simulink library "TerryBodyBlockLib2G"  (R2018a)
settings: Solver=ode45  StartTime=0.0  StopTime=10.0  RelTol=1e-3  EnableMultiTasking=on
undefined symbols (not defined in the file): BaseMass, E, ExtendedActuatorLength, FollowerMass, H, L, N, rho, W, X, Y, Z
libraries: sm_lib x270, nesl_utility x94, fl_lib x18, simulink x2
(part 1 of 6)
settings Model: Creator=tdenery  LastModifiedBy=tdenery
settings DataIOCC: LimitDataPoints=on  SaveFormat=Array  SignalLoggingSaveFormat=ModelDataLogs
settings OptimizationCC: ExpressionDepthLimit=2147483647  LifeSpan=inf
settings DebuggingCC: UnderspecifiedInitializationDetection=Classic  MergeDetectMultiDrivingBlocksExec=none  SolverPrmCheckMsg=warning  FcnCallInpInsideContextMsg=warning  StateNameClashWarn=warning  SFUnexpectedBacktrackingDiag=warning  SFNoUnconditionalDefaultTransitionDiag=warning  SFExecutionAtInitializationDiag=none
settings HardwareCC: ProdBitPerPointer=32  ProdBitPerSizeT=32  ProdBitPerPtrDiffT=32  ProdLargestAtomicFloat=None  ProdIntDivRoundTo=Undefined  ProdEndianess=Unspecified  ProdWordSize=32  ProdHWDeviceType=32-bit Generic
settings ModelReferenceCC: PropagateSignalLabelsOutOfModel=off
settings CodeAppCC: StateflowObjectComments=on
settings GRTTargetCC: TargetLangStandard=C89/C90 (ANSI)  GeneratePreprocessorConditionals=Disable all  CombineOutputUpdateFcns=off  GRTInterface=on
settings ConfigComp: CovMetricSettings=dw  CovHtmlReporting=on  CovSaveCumulativeToWorkspaceVar=on  CovSaveSingleToWorkspaceVar=on  CovExternalEMLEnable=off  CovSFcnEnable=off

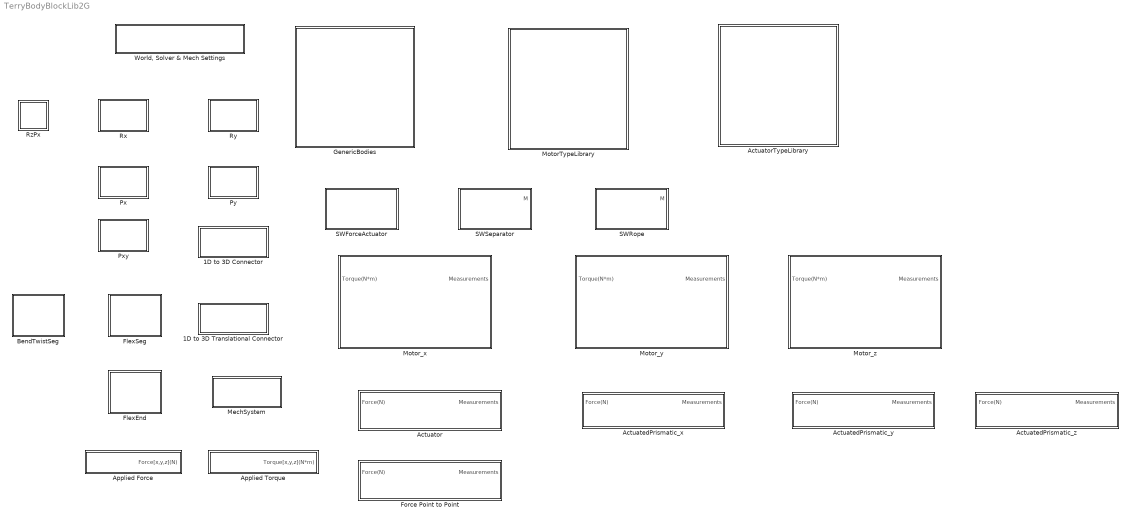
== system TerryBodyBlockLib2G ==
  1D to 3D Connector : Subsystem
  1D to 3D Translational Connector : Subsystem  Tag=Mech1D3DConverter
  ActuatedPrismatic_x : Subsystem  Tag=Force  mask{ActuationType=Force}
      mask prompts: ActuationType "Actuation Type"
      mask TypeOptions ActuationType: Motion | Force | Shaft
      mask Callback ActuationType:
      | maskStr = get_param( gcb, 'ActuationType' );
      | ActuatorBlockHandle = gcbh;
      | ActuatorBlockSystemName = [get_param( ActuatorBlockHandle, 'Parent' ), '/', get_param( ActuatorBlockHandle, 'Name' )];
      | CurrentConfig = get_param( ActuatorBlockHandle, 'Tag' );
      | if ~strcmp( maskStr, CurrentConfig )
      |     hInport = find_system(ActuatorBlockHandle,'LookUnderMasks','all','SearchDepth','1','BlockType','Inport');
      |     if ~isempty( hInport )
      |         hPH = get_param( hInport, 'PortHandles' );
      |         PortPosition = get_param( hInport, 'Position' );
      |         PortPositionStringForSetParam = ['[', num2str( PortPosition(1) ), ', ', num2str( PortPosition(2) ), ', ', num2str( PortPosition(3) ), ', ', num2str( PortPosition(4) ), ']'];
      |         hLine = get_param( hPH.Outport, 'Line' );
      |         delete_block( hInport );
      |         delete( hLine );
      |     end
      |     hExternalPort = find_system(ActuatorBlockHandle,'LookUnderMasks','all','Name','ActuatorShaft');
      |     if ~isempty( hExternalPort )
      |         hPH = get_param( hExternalPort, 'PortHandles' );
      |         PortPosition = get_param( hExternalPort, 'Position' );
      |         PortPositionStringForSetParam = ['[', num2str( PortPosition(1) ), ', ', num2str( PortPosition(2) ), ', ', num2str( PortPosition(3) ), ', ', num2str( PortPosition(4) ), ']'];
      |         hLine = get_param( hPH.RConn, 'Line' );
      |         delete_block( hExternalPort );
      |         delete( hLine );
      |     end
      |     hActuatorBlock = find_system(ActuatorBlockHandle,'LookUnderMasks','all','Tag','Actuator');
      |     BlockPos = get_param( hActuatorBlock, 'Position' );
      |     ActuatorPositionStringForSetParam = ['[', num2str( BlockPos(1) ), ', ', num2str( BlockPos(2) ), ', ', num2str( BlockPos(3) ), ', ', num2str( BlockPos(4) ), ']'];
      |     delete_block( hActuatorBlock );
      | 
      |     if strcmpi(maskStr, 'Force')
      |         hActuatorBlock = add_block( 'TerryBodyBlockLib2G/ActuatorTypeLibrary/ForceActuatedPrismatic', [ActuatorBlockSystemName, '/ForceActuator'] );
      |         set_param( hActuatorBlock, 'LinkStatus', 'none' );
      |         set_param( ActuatorBlockHandle, 'Tag', 'Force' );
      |         set_param( hActuatorBlock, 'Position', ActuatorPositionStringForSetParam );
      |         hInport = add_block( 'simulink/Sources/In1', [ActuatorBlockSystemName, '/Force(N)'] );
      |         set_param( hInport, 'Position', PortPositionStringForSetParam );
      |         hInportHandles = get_param( hInport, 'PortHandles' );
      |         hActuatorPortHandles = get_param( hActuatorBlock, 'PortHandles' );
      |         add_line(ActuatorBlockSystemName,hInportHandles.Outport(1),hActuatorPortHandles.Inport(1));
      |     elseif strcmpi(maskStr, 'Motion')
      |         hActuatorBlock = add_block( 'TerryBodyBlockLib2G/ActuatorTypeLibrary/MotionActuatedPrismatic', [ActuatorBlockSystemName, '/MotionActuator'] );
      |         set_param( hActuatorBlock, 'LinkStatus', 'none' );
      |         set_param( ActuatorBlockHandle, 'Tag', 'Motion' );
      |         set_param( hActuatorBlock, 'Position', ActuatorPositionStringForSetParam );
      |         hInport = add_block( 'simulink/Sources/In1', [ActuatorBlockSystemName, '/Motion( pva, m, s )'] );
      |         set_param( hInport, 'Position', PortPositionStringForSetParam );
      |         hInportHandles = get_param( hInport, 'PortHandles' );
      |         hActuatorPortHandles = get_param( hActuatorBlock, 'PortHandles' );
      |         add_line(ActuatorBlockSystemName,hInportHandles.Outport(1),hActuatorPortHandles.Inport(1));
      |     elseif strcmpi(maskStr, 'Shaft')
      |         hActuatorBlock = add_block( 'TerryBodyBlockLib2G/ActuatorTypeLibrary/ShaftActuatedPrismatic', [ActuatorBlockSystemName, '/ShaftMotor'] );
      |         set_param( hActuatorBlock, 'LinkStatus', 'none' );
      |         set_param( ActuatorBlockHandle, 'Tag', 'Shaft' );
      |         set_param( hActuatorBlock, 'Position', ActuatorPositionStringForSetParam );
      |         hExternalPort = add_block( 'nesl_utility/Connection Port', [ActuatorBlockSystemName, '/ActuatorShaft'] );
      |         set_param( hExternalPort, 'Port', '1' );
      |         set_param( hExternalPort, 'Side', 'Left' );
      |         set_param( hExternalPort, 'Position', PortPositionStringForSetParam );
      |         hExPortHandles = get_param( hExternalPort, 'PortHandles' );
      |         hActuatorPortHandles = get_param( hActuatorBlock, 'PortHandles' );
      |         add_line(ActuatorBlockSystemName,hExPortHandles.RConn(1),hActuatorPortHandles.LConn(1));
      |     end
      | end
      | clear( 'BlockPos', 'CurrentConfig', 'hExPortHandles', 'hExternalPort', 'hInport', 'hInportHandles', 'hLine', 'hActuatorBlock', 'hActuatorPortHandles', 'hPH', 'maskStr', 'ActuatorBlockHandle', 'ActuatorBlockSystemName', 'ActuatorPositionStringForSetParam', 'PortPosition', 'PortPositionStringForSetParam' );
  ActuatedPrismatic_y : Subsystem  Tag=Force  mask{ActuationType=Force}
      mask prompts: ActuationType "Actuation Type"
      mask TypeOptions ActuationType: Motion | Force | Shaft
      mask Callback ActuationType:
      | maskStr = get_param( gcb, 'ActuationType' );
      | ActuatorBlockHandle = gcbh;
      | ActuatorBlockSystemName = [get_param( ActuatorBlockHandle, 'Parent' ), '/', get_param( ActuatorBlockHandle, 'Name' )];
      | CurrentConfig = get_param( ActuatorBlockHandle, 'Tag' );
      | if ~strcmp( maskStr, CurrentConfig )
      |     hInport = find_system(ActuatorBlockHandle,'LookUnderMasks','all','SearchDepth','1','BlockType','Inport');
      |     if ~isempty( hInport )
      |         hPH = get_param( hInport, 'PortHandles' );
      |         PortPosition = get_param( hInport, 'Position' );
      |         PortPositionStringForSetParam = ['[', num2str( PortPosition(1) ), ', ', num2str( PortPosition(2) ), ', ', num2str( PortPosition(3) ), ', ', num2str( PortPosition(4) ), ']'];
      |         hLine = get_param( hPH.Outport, 'Line' );
      |         delete_block( hInport );
      |         delete( hLine );
      |     end
      |     hExternalPort = find_system(ActuatorBlockHandle,'LookUnderMasks','all','Name','ActuatorShaft');
      |     if ~isempty( hExternalPort )
      |         hPH = get_param( hExternalPort, 'PortHandles' );
      |         PortPosition = get_param( hExternalPort, 'Position' );
      |         PortPositionStringForSetParam = ['[', num2str( PortPosition(1) ), ', ', num2str( PortPosition(2) ), ', ', num2str( PortPosition(3) ), ', ', num2str( PortPosition(4) ), ']'];
      |         hLine = get_param( hPH.RConn, 'Line' );
      |         delete_block( hExternalPort );
      |         delete( hLine );
      |     end
      |     hActuatorBlock = find_system(ActuatorBlockHandle,'LookUnderMasks','all','Tag','Actuator');
      |     BlockPos = get_param( hActuatorBlock, 'Position' );
      |     ActuatorPositionStringForSetParam = ['[', num2str( BlockPos(1) ), ', ', num2str( BlockPos(2) ), ', ', num2str( BlockPos(3) ), ', ', num2str( BlockPos(4) ), ']'];
      |     delete_block( hActuatorBlock );
      | 
      |     if strcmpi(maskStr, 'Force')
      |         hActuatorBlock = add_block( 'TerryBodyBlockLib2G/ActuatorTypeLibrary/ForceActuatedPrismatic', [ActuatorBlockSystemName, '/ForceActuator'] );
      |         set_param( hActuatorBlock, 'LinkStatus', 'none' );
      |         set_param( ActuatorBlockHandle, 'Tag', 'Force' );
      |         set_param( hActuatorBlock, 'Position', ActuatorPositionStringForSetParam );
      |         hInport = add_block( 'simulink/Sources/In1', [ActuatorBlockSystemName, '/Force(N)'] );
      |         set_param( hInport, 'Position', PortPositionStringForSetParam );
      |         hInportHandles = get_param( hInport, 'PortHandles' );
      |         hActuatorPortHandles = get_param( hActuatorBlock, 'PortHandles' );
      |         add_line(ActuatorBlockSystemName,hInportHandles.Outport(1),hActuatorPortHandles.Inport(1));
      |     elseif strcmpi(maskStr, 'Motion')
      |         hActuatorBlock = add_block( 'TerryBodyBlockLib2G/ActuatorTypeLibrary/MotionActuatedPrismatic', [ActuatorBlockSystemName, '/MotionActuator'] );
      |         set_param( hActuatorBlock, 'LinkStatus', 'none' );
      |         set_param( ActuatorBlockHandle, 'Tag', 'Motion' );
      |         set_param( hActuatorBlock, 'Position', ActuatorPositionStringForSetParam );
      |         hInport = add_block( 'simulink/Sources/In1', [ActuatorBlockSystemName, '/Motion( pva, m, s )'] );
      |         set_param( hInport, 'Position', PortPositionStringForSetParam );
      |         hInportHandles = get_param( hInport, 'PortHandles' );
      |         hActuatorPortHandles = get_param( hActuatorBlock, 'PortHandles' );
      |         add_line(ActuatorBlockSystemName,hInportHandles.Outport(1),hActuatorPortHandles.Inport(1));
      |     elseif strcmpi(maskStr, 'Shaft')
      |         hActuatorBlock = add_block( 'TerryBodyBlockLib2G/ActuatorTypeLibrary/ShaftActuatedPrismatic', [ActuatorBlockSystemName, '/ShaftMotor'] );
      |         set_param( hActuatorBlock, 'LinkStatus', 'none' );
      |         set_param( ActuatorBlockHandle, 'Tag', 'Shaft' );
      |         set_param( hActuatorBlock, 'Position', ActuatorPositionStringForSetParam );
      |         hExternalPort = add_block( 'nesl_utility/Connection Port', [ActuatorBlockSystemName, '/ActuatorShaft'] );
      |         set_param( hExternalPort, 'Port', '1' );
      |         set_param( hExternalPort, 'Side', 'Left' );
      |         set_param( hExternalPort, 'Position', PortPositionStringForSetParam );
      |         hExPortHandles = get_param( hExternalPort, 'PortHandles' );
      |         hActuatorPortHandles = get_param( hActuatorBlock, 'PortHandles' );
      |         add_line(ActuatorBlockSystemName,hExPortHandles.RConn(1),hActuatorPortHandles.LConn(1));
      |     end
      | end
      | clear( 'BlockPos', 'CurrentConfig', 'hExPortHandles', 'hExternalPort', 'hInport', 'hInportHandles', 'hLine', 'hActuatorBlock', 'hActuatorPortHandles', 'hPH', 'maskStr', 'ActuatorBlockHandle', 'ActuatorBlockSystemName', 'ActuatorPositionStringForSetParam', 'PortPosition', 'PortPositionStringForSetParam' );
  ActuatedPrismatic_z : Subsystem  Tag=Force  mask{ActuationType=Force}
      mask prompts: ActuationType "Actuation Type"
      mask TypeOptions ActuationType: Motion | Force | Shaft
      mask Callback ActuationType:
      | maskStr = get_param( gcb, 'ActuationType' );
      | ActuatorBlockHandle = gcbh;
      | ActuatorBlockSystemName = [get_param( ActuatorBlockHandle, 'Parent' ), '/', get_param( ActuatorBlockHandle, 'Name' )];
      | CurrentConfig = get_param( ActuatorBlockHandle, 'Tag' );
      | if ~strcmp( maskStr, CurrentConfig )
      |     hInport = find_system(ActuatorBlockHandle,'LookUnderMasks','all','SearchDepth','1','BlockType','Inport');
      |     if ~isempty( hInport )
      |         hPH = get_param( hInport, 'PortHandles' );
      |         PortPosition = get_param( hInport, 'Position' );
      |         PortPositionStringForSetParam = ['[', num2str( PortPosition(1) ), ', ', num2str( PortPosition(2) ), ', ', num2str( PortPosition(3) ), ', ', num2str( PortPosition(4) ), ']'];
      |         hLine = get_param( hPH.Outport, 'Line' );
      |         delete_block( hInport );
      |         delete( hLine );
      |     end
      |     hExternalPort = find_system(ActuatorBlockHandle,'LookUnderMasks','all','Name','ActuatorShaft');
      |     if ~isempty( hExternalPort )
      |         hPH = get_param( hExternalPort, 'PortHandles' );
      |         PortPosition = get_param( hExternalPort, 'Position' );
      |         PortPositionStringForSetParam = ['[', num2str( PortPosition(1) ), ', ', num2str( PortPosition(2) ), ', ', num2str( PortPosition(3) ), ', ', num2str( PortPosition(4) ), ']'];
      |         hLine = get_param( hPH.RConn, 'Line' );
      |         delete_block( hExternalPort );
      |         delete( hLine );
      |     end
      |     hActuatorBlock = find_system(ActuatorBlockHandle,'LookUnderMasks','all','Tag','Actuator');
      |     BlockPos = get_param( hActuatorBlock, 'Position' );
      |     ActuatorPositionStringForSetParam = ['[', num2str( BlockPos(1) ), ', ', num2str( BlockPos(2) ), ', ', num2str( BlockPos(3) ), ', ', num2str( BlockPos(4) ), ']'];
      |     delete_block( hActuatorBlock );
      | 
      |     if strcmpi(maskStr, 'Force')
      |         hActuatorBlock = add_block( 'TerryBodyBlockLib2G/ActuatorTypeLibrary/ForceActuatedPrismatic', [ActuatorBlockSystemName, '/ForceActuator'] );
      |         set_param( hActuatorBlock, 'LinkStatus', 'none' );
      |         set_param( ActuatorBlockHandle, 'Tag', 'Force' );
      |         set_param( hActuatorBlock, 'Position', ActuatorPositionStringForSetParam );
      |         hInport = add_block( 'simulink/Sources/In1', [ActuatorBlockSystemName, '/Force(N)'] );
      |         set_param( hInport, 'Position', PortPositionStringForSetParam );
      |         hInportHandles = get_param( hInport, 'PortHandles' );
      |         hActuatorPortHandles = get_param( hActuatorBlock, 'PortHandles' );
      |         add_line(ActuatorBlockSystemName,hInportHandles.Outport(1),hActuatorPortHandles.Inport(1));
      |     elseif strcmpi(maskStr, 'Motion')
      |         hActuatorBlock = add_block( 'TerryBodyBlockLib2G/ActuatorTypeLibrary/MotionActuatedPrismatic', [ActuatorBlockSystemName, '/MotionActuator'] );
      |         set_param( hActuatorBlock, 'LinkStatus', 'none' );
      |         set_param( ActuatorBlockHandle, 'Tag', 'Motion' );
      |         set_param( hActuatorBlock, 'Position', ActuatorPositionStringForSetParam );
      |         hInport = add_block( 'simulink/Sources/In1', [ActuatorBlockSystemName, '/Motion( pva, m, s )'] );
      |         set_param( hInport, 'Position', PortPositionStringForSetParam );
      |         hInportHandles = get_param( hInport, 'PortHandles' );
      |         hActuatorPortHandles = get_param( hActuatorBlock, 'PortHandles' );
      |         add_line(ActuatorBlockSystemName,hInportHandles.Outport(1),hActuatorPortHandles.Inport(1));
      |     elseif strcmpi(maskStr, 'Shaft')
      |         hActuatorBlock = add_block( 'TerryBodyBlockLib2G/ActuatorTypeLibrary/ShaftActuatedPrismatic', [ActuatorBlockSystemName, '/ShaftMotor'] );
      |         set_param( hActuatorBlock, 'LinkStatus', 'none' );
      |         set_param( ActuatorBlockHandle, 'Tag', 'Shaft' );
      |         set_param( hActuatorBlock, 'Position', ActuatorPositionStringForSetParam );
      |         hExternalPort = add_block( 'nesl_utility/Connection Port', [ActuatorBlockSystemName, '/ActuatorShaft'] );
      |         set_param( hExternalPort, 'Port', '1' );
      |         set_param( hExternalPort, 'Side', 'Left' );
      |         set_param( hExternalPort, 'Position', PortPositionStringForSetParam );
      |         hExPortHandles = get_param( hExternalPort, 'PortHandles' );
      |         hActuatorPortHandles = get_param( hActuatorBlock, 'PortHandles' );
      |         add_line(ActuatorBlockSystemName,hExPortHandles.RConn(1),hActuatorPortHandles.LConn(1));
      |     end
      | end
      | clear( 'BlockPos', 'CurrentConfig', 'hExPortHandles', 'hExternalPort', 'hInport', 'hInportHandles', 'hLine', 'hActuatorBlock', 'hActuatorPortHandles', 'hPH', 'maskStr', 'ActuatorBlockHandle', 'ActuatorBlockSystemName', 'ActuatorPositionStringForSetParam', 'PortPosition', 'PortPositionStringForSetParam' );
  Actuator : Subsystem  Tag=Force  mask{ActuationType=Force, InitialActuatorLength=1.869564, ActuatorMass=0.1}
      mask prompts: ActuationType "Actuation Type"; InitialActuatorLength "Initial Length (m)"; ActuatorMass "Actuator Mass (kg)"
      mask init:
      | ExtendedActuatorLength = InitialActuatorLength*4/3;
      | ActuatorBaseRadius = ExtendedActuatorLength/20;
      | ActuatorFollowerRadius = ExtendedActuatorLength/25;
      | AreaBaseCrossSection = pi*ActuatorBaseRadius^2;
      | AreaFollowerCrossSection = pi*ActuatorFollowerRadius^2;
      | BaseVolume = ExtendedActuatorLength*AreaBaseCrossSection;
      | FollowerVolume = ExtendedActuatorLength*AreaFollowerCrossSection;
      | TotalVolume = BaseVolume + FollowerVolume;
      | BaseMass = ActuatorMass*BaseVolume/TotalVolume;
      | FollowerMass = ActuatorMass*FollowerVolume/TotalVolume;
      mask TypeOptions ActuationType: Motion | Force | Shaft
      mask Callback ActuationType:
      | maskStr = get_param( gcb, 'ActuationType' );
      | ActuatorBlockHandle = gcbh;
      | ActuatorBlockSystemName = [get_param( ActuatorBlockHandle, 'Parent' ), '/', get_param( ActuatorBlockHandle, 'Name' )];
      | CurrentConfig = get_param( ActuatorBlockHandle, 'Tag' );
      | if ~strcmp( maskStr, CurrentConfig )
      |     hInport = find_system(ActuatorBlockHandle,'LookUnderMasks','all','SearchDepth','1','BlockType','Inport');
      |     if ~isempty( hInport )
      |         hPH = get_param( hInport, 'PortHandles' );
      |         PortPosition = get_param( hInport, 'Position' );
      |         PortPositionStringForSetParam = ['[', num2str( PortPosition(1) ), ', ', num2str( PortPosition(2) ), ', ', num2str( PortPosition(3) ), ', ', num2str( PortPosition(4) ), ']'];
      |         hLine = get_param( hPH.Outport, 'Line' );
      |         delete_block( hInport );
      |         delete( hLine );
      |     end
      |     hExternalPort = find_system(ActuatorBlockHandle,'LookUnderMasks','all','Name','ActuatorShaft');
      |     if ~isempty( hExternalPort )
      |         hPH = get_param( hExternalPort, 'PortHandles' );
      |         PortPosition = get_param( hExternalPort, 'Position' );
      |         PortPositionStringForSetParam = ['[', num2str( PortPosition(1) ), ', ', num2str( PortPosition(2) ), ', ', num2str( PortPosition(3) ), ', ', num2str( PortPosition(4) ), ']'];
      |         hLine = get_param( hPH.RConn, 'Line' );
      |         delete_block( hExternalPort );
      |         delete( hLine );
      |     end
      |     hActuatorBlock = find_system(ActuatorBlockHandle,'LookUnderMasks','all','Tag','Actuator');
      |     BlockPos = get_param( hActuatorBlock, 'Position' );
      |     ActuatorPositionStringForSetParam = ['[', num2str( BlockPos(1) ), ', ', num2str( BlockPos(2) ), ', ', num2str( BlockPos(3) ), ', ', num2str( BlockPos(4) ), ']'];
      | %     hInitTransform = find_system(ActuatorBlockHandle,'LookUnderMasks','all','Name','TransformThatSetsF');
      | %     TransformThatSetsF_Angle = get_param( hInitTransform, 'RotationAngle' );
      | %     TransformThatSetsF_Axis = get_param( hInitTransform, 'RotationArbitraryAxis' );
      | %     hUJoint = find_system(ActuatorBlockHandle,'LookUnderMasks','all','Name','RevXFor_ExtensionActuator');
      | %     InitialSetUJoint_RxPosition = get_param( hUJoint, 'RxPositionTargetValue' );
      |     delete_block( hActuatorBlock );
      | 
      |     if strcmpi(maskStr, 'Force')
      |         hActuatorBlock = add_block( 'TerryBodyBlockLib2G/ActuatorTypeLibrary/ForceActuatedPrismatic', [ActuatorBlockSystemName, '/ForceActuator'] );
      |         set_param( hActuatorBlock, 'LinkStatus', 'none' );
      |         set_param( ActuatorBlockHandle, 'Tag', 'Force' );
      |         set_param( hActuatorBlock, 'Position', ActuatorPositionStringForSetParam );
      |         hInport = add_block( 'simulink/Sources/In1', [ActuatorBlockSystemName, '/Force(N)'] );
      |         set_param( hInport, 'Position', PortPositionStringForSetParam );
      |         hInportHandles = get_param( hInport, 'PortHandles' );
      |         hActuatorPortHandles = get_param( hActuatorBlock, 'PortHandles' );
      |         add_line(ActuatorBlockSystemName,hInportHandles.Outport(1),hActuatorPortHandles.Inport(1));
      |     elseif strcmpi(maskStr, 'Motion')
      |         hActuatorBlock = add_block( 'TerryBodyBlockLib2G/ActuatorTypeLibrary/MotionActuatedPrismatic', [ActuatorBlockSystemName, '/MotionActuator'] );
      |         set_param( hActuatorBlock, 'LinkStatus', 'none' );
      |         set_param( ActuatorBlockHandle, 'Tag', 'Motion' );
      |         set_param( hActuatorBlock, 'Position', ActuatorPositionStringForSetParam );
      |         hInport = add_block( 'simulink/Sources/In1', [ActuatorBlockSystemName, '/Motion( pva, m, s )'] );
      |         set_param( hInport, 'Position', PortPositionStringForSetParam );
      |         hInportHandles = get_param( hInport, 'PortHandles' );
      |         hActuatorPortHandles = get_param( hActuatorBlock, 'PortHandles' );
      |         add_line(ActuatorBlockSystemName,hInportHandles.Outport(1),hActuatorPortHandles.Inport(1));
      |     elseif strcmpi(maskStr, 'Shaft')
      |         hActuatorBlock = add_block( 'TerryBodyBlockLib2G/ActuatorTypeLibrary/ShaftActuatedPrismatic', [ActuatorBlockSystemName, '/ShaftMotor'] );
      |         set_param( hActuatorBlock, 'LinkStatus', 'none' );
      |         set_param( ActuatorBlockHandle, 'Tag', 'Shaft' );
      |         set_param( hActuatorBlock, 'Position', ActuatorPositionStringForSetParam );
      |         hExternalPort = add_block( 'nesl_utility/Connection Port', [ActuatorBlockSystemName, '/ActuatorShaft'] );
      |         set_param( hExternalPort, 'Port', '1' );
      |         set_param( hExternalPort, 'Side', 'Left' );
      |         set_param( hExternalPort, 'Position', PortPositionStringForSetParam );
      |         hExPortHandles = get_param( hExternalPort, 'PortHandles' );
      |         hActuatorPortHandles = get_param( hActuatorBlock, 'PortHandles' );
      |         add_line(ActuatorBlockSystemName,hExPortHandles.RConn(1),hActuatorPortHandles.LConn(1));
      |     end
      | %     hInitTransform = find_system(ActuatorBlockHandle,'LookUnderMasks','all','Name','TransformThatSetsF');
      | %     set_param( hInitTransform, 'RotationAngle', TransformThatSetsF_Angle );
      | %     set_param( hInitTransform, 'RotationArbitraryAxis', TransformThatSetsF_Axis );
      | %     hUJoint = find_system(ActuatorBlockHandle,'LookUnderMasks','all','Name','RevXFor_ExtensionActuator');
      | %     InitialSetUJoint_RxPosition = set_param( hUJoint, 'RxPositionTargetValue', InitialSetUJoint_RxPosition );
      | end
      | clear( 'BlockPos', 'CurrentConfig', 'hExPortHandles', 'hExternalPort', 'hInport', 'hInportHandles', 'hLine', 'hActuatorBlock', 'hActuatorPortHandles', 'hPH', 'maskStr', 'ActuatorBlockHandle', 'ActuatorBlockSystemName', 'ActuatorPositionStringForSetParam', 'PortPosition', 'PortPositionStringForSetParam' );
  ActuatorTypeLibrary : Subsystem
  Applied Force : Subsystem  mask(Applied Force){}
      mask help:
      | Receives a 3-component signal and applies it to a SimMechanics body as a 3-dimensional force.  The input signal 1,2,3 - elements map to x,y,z components of a force vector resolved in the frame of the attached coordinate system.
      |
      | The units for force are Newtons.
  Applied Torque : Subsystem  mask(Applied Force){}
      mask help:
      | Receives a 3-component signal and applies it to a SimMechanics body as a 3-dimensional torque.  The input signal 1,2,3 - elements map to x,y,z components of a torque vector resolved in the frame of the attached coordinate system.
      |
      | The units for force are Newton*meters.
  BendTwistSeg : Subsystem  mask{E=E, rho=rho, x=L/N, y=W, z=H}
      mask prompts: E "Modulus of Elasticity (Pa)"; rho "Mass Density (kg/m^3)"; x "Length[x] (m)"; y "Width[y] (m)"; z "Height [z] (m)"
      mask init:
      | Izz = z*y^3/12;
      | Iyy = y*z^3/12;
      | ky = Iyy*E/x;
      | kz = Izz*E/x;
      | if y > z
      |     a = y;
      |     b = z;
      | else
      |     a = z;
      |     b = y;
      | end
      | J = a*b^3*(1/3 -0.21*b/a*( 1 - b^4/12/a^4));
      | nu = 0.4; %Poisson's Ratio
      | G = E/2/(1+nu);
      | k_theta = G*J/x;
  FlexEnd : Subsystem  mask{E=E, rho=rho, x=L/N, y=W, z=H}
      mask prompts: E "Modulus of Elasticity (Pa)"; rho "Mass Density (kg/m^3)"; x "Length[x] (m)"; y "Width[y] (m)"; z "Height [z] (m)"
      mask init:
      | Izz = z*y^3/12;
      | Iyy = y*z^3/12;
      | ky = Iyy*E/x;
      | kz = Izz*E/x;
  FlexSeg : Subsystem  mask{E=E, rho=rho, x=L/N, y=W, z=H}
      mask prompts: E "Modulus of Elasticity (Pa)"; rho "Mass Density (kg/m^3)"; x "Length[x] (m)"; y "Width[y] (m)"; z "Height [z] (m)"
      mask init:
      | Izz = z*y^3/12;
      | Iyy = y*z^3/12;
      | ky = Iyy*E/x;
      | kz = Izz*E/x;
      | if y > z
      |     a = y;
      |     b = z;
      | else
      |     a = z;
      |     b = y;
      | end
      | J = a*b^3(1/3 -0.21*b/a*( 1 - b^4/12/a^4));
      | nu = 0.4; %Poisson's Ratio
      | G = E/2/(1+nu);
      | k_theta = G*J/x;
  Force Point to Point : Subsystem
  GenericBodies : Subsystem
  MechSystem : Subsystem  mask{PopupParam=Force/Torque}
      mask prompts: PopupParam "Motion Configuration"
      mask TypeOptions PopupParam: Force/Torque | Motion
      mask Callback PopupParam:
      | MechSystem = gcb;
      | MotionConfig = get_param( MechSystem, 'PopupParam' );
      | CurrentConfig = get_param( MechSystem, 'Tag' );
      | if ~strcmp( MotionConfig, CurrentConfig )
      |     MotOutports = find_system(MechSystem,'LookUnderMasks','all','Tag','MechSystemMotorOutport');
      |     ActOutports = find_system(MechSystem,'LookUnderMasks','all','Tag','MechSystemActuatorOutport');
      |     APOutports = find_system(MechSystem,'LookUnderMasks','all','Tag','MechSystemAPOutport');
      |     NMotors = length( MotOutports );
      |     NActuators = length( ActOutports );
      |     NActuatedPrismatics = length( APOutports );
      |     if NMotors > 0
      |         hMotOutports( NMotors ) = 0;
      |         hMotors( NMotors ) = 0;
      |         hMotInports( NMotors ) = 0;
      |         MotNameRoot{NMotors} = '';
      |     end
      |     if NActuators > 0
      |         hActOutports( NActuators ) = 0;
      |         hActuators( NActuators ) = 0;
      |         hActInports( NActuators ) = 0;
      |         ActNameRoot{NActuators} = '';
      |     end
      |     if NActuatedPrismatics > 0
      |         hAPOutports( NActuatedPrismatics ) = 0;
      |         hActuatedPrismatics( NActuatedPrismatics ) = 0;
      |         hAPInports( NActuatedPrismatics ) = 0;
      |         APNameRoot{NActuatedPrismatics} = '';
      |     end
      | 
      |     for i = 1:NMotors
      |         hMotOutports(i) = getSimulinkBlockHandle( MotOutports(i) );
      |         OutportName = get_param( hMotOutports(i), 'Name' );
      |         NameLength = length( OutportName );
      |         MotNameRoot{i} = OutportName( 1:NameLength-2 );
      |         hP = get_param( hMotOutports(i), 'PortHandles' );
      |         hL = get_param( hP.Inport, 'Line' );
      |         hMotors(i) = get_param( hL, 'SrcBlockHandle' );
      |         hpMotor(i) = get_param( hMotors(i), 'PortHandles' );
      |     end
      |     for i = 1:NActuators
      |         hActOutports(i) = getSimulinkBlockHandle( ActOutports(i) );
      |         OutportName = get_param( hActOutports(i), 'Name' );
      |         NameLength = length( OutportName );
      |         ActNameRoot{i} = OutportName( 1:NameLength-2 );
      |         hP = get_param( hActOutports(i), 'PortHandles' );
      |         hL = get_param( hP.Inport, 'Line' );
      |         hActuators(i) = get_param( hL, 'SrcBlockHandle' );
      |         hpActuator(i) = get_param( hActuators(i), 'PortHandles' );
      |     end
      |     for i = 1:NActuatedPrismatics
      |         hAPOutports(i) = getSimulinkBlockHandle( APOutports(i) );
      |         OutportName = get_param( hAPOutports(i), 'Name' );
      |         NameLength = length( OutportName );
      |         APNameRoot{i} = OutportName( 1:NameLength-2 );
      |         hP = get_param( hAPOutports(i), 'PortHandles' );
      |         hL = get_param( hP.Inport, 'Line' );
      |         hActuatedPrismatics(i) = get_param( hL, 'SrcBlockHandle' );
      |         hpActuatedPrismatic(i) = get_param( hActuatedPrismatics(i), 'PortHandles' );
      |     end
      | 
      |     if strcmp( MotionConfig, 'Force/Torque' ) || strcmp( MotionConfig, 'Motion' )
      | 
      |         for i = 1:NMotors
      |             if isempty( hpMotor(i).Inport )
      |                 hMotInports(i) = add_block( 'simulink/Sources/In1', [MechSystem, '/Fred', num2str(i)] );
      |                 OutPos = get_param( MotOutports(i), 'Position' );
      |                 InPos = OutPos{1} + [-300, 0, -300, 0];
      |                 set_param( hMotInports(i), 'Position', ['[', num2str(InPos(1)), ',', num2str(InPos(2)), ',', num2str(InPos(3)), ',', num2str(InPos(4)), ']'] );
      |                 set_param( hMotInports(i), 'Tag', 'MechSystemMotorInport' );
      |             else
      |                 hP = hpMotor(i).Inport;
      |                 hL = get_param( hP, 'Line' );
      |                 hMotInports(i) = get_param( hL, 'SrcBlockHandle' );
      |             end
      |         end
      |         for i = 1:NActuators
      |             if isempty( hpActuator(i).Inport )
      |                 hActInports(i) = add_block( 'simulink/Sources/In1', [MechSystem, '/Fred', num2str(i)] );
      |                 OutPos = get_param( ActOutports(i), 'Position' );
      |                 InPos = OutPos{1} + [-300, 0, -300, 0];
      |                 set_param( hActInports(i), 'Position', ['[', num2str(InPos(1)), ',', num2str(InPos(2)), ',', num2str(InPos(3)), ',', num2str(InPos(4)), ']'] );
      |                 set_param( hActInports(i), 'Tag', 'MechSystemACtuatorInport' );
      |             else
      |                 hP = hpActuator(i).Inport;
      |                 hL = get_param( hP, 'Line' );
      |                 hActInports(i) = get_param( hL, 'SrcBlockHandle' );
      |             end
      |         end
      |         for i = 1:NActuatedPrismatics
      |             if isempty( hpActuatedPrismatic(i).Inport )
      |                 hAPInports(i) = add_block( 'simulink/Sources/In1', [MechSystem, '/Fred', num2str(i)] );
      |                 OutPos = get_param( APOutports(i), 'Position' );
      |                 InPos = OutPos{1} + [-300, 0, -300, 0];
      |                 set_param( hAPInports(i), 'Position', ['[', num2str(InPos(1)), ',', num2str(InPos(2)), ',', num2str(InPos(3)), ',', num2str(InPos(4)), ']'] );
      |                 set_param( hAPInports(i), 'Tag', 'MechSystemACtuatorInport' );
      |             else
      |                 hP = hpActuatedPrismatic(i).Inport;
      |                 hL = get_param( hP, 'Line' );
      |                 hAPInports(i) = get_param( hL, 'SrcBlockHandle' );
      |             end
      |         end
      | 
      |         if strcmp( MotionConfig, 'Force/Torque' )
      |             set_param( MechSystem, 'Tag', 'Force/Torque' );
      |             for i = 1:NMotors
      |                 o = get_param( hMotors(i), 'Object' );
      |                 o.MotorType = 'Torque';
      |                 set_param( hMotInports(i), 'Name', [MotNameRoot{i}, '(N*m)'] );
      |                 hP = get_param( hMotInports(i), 'PortHandles' );
      |                 hL = get_param( hP.Outport, 'Line' );
      |                 if hL ~= -1
      |                     delete_line( hL );
      |                 end
      |                 add_line( MechSystem, [get_param( hMotInports(i), 'Name' ), '/1'], [get_param( hMotors(i), 'Name' ), '/1'] );
      |             end
      |             for i = 1:NActuators
      |                 o = get_param( hActuators(i), 'Object' );
      |                 o.ActuationType = 'Force';
      |                 set_param( hActInports(i), 'Name', [ActNameRoot{i}, '(N)'] );
      |                 hP = get_param( hActInports(i), 'PortHandles' );
      |                 hL = get_param( hP.Outport, 'Line' );
      |                 if hL ~= -1
      |                     delete_line( hL );
      |                 end
      |                 add_line( MechSystem, [get_param( hActInports(i), 'Name' ), '/1'], [get_param( hActuators(i), 'Name' ), '/1'] );
      |             end
      |             for i = 1:NActuatedPrismatics
      |                 o = get_param( hActuatedPrismatics(i), 'Object' );
      |                 o.ActuationType = 'Force';
      |                 set_param( hAPInports(i), 'Name', [APNameRoot{i}, '(N)'] );
      |                 hP = get_param( hAPInports(i), 'PortHandles' );
      |                 hL = get_param( hP.Outport, 'Line' );
      |                 if hL ~= -1
      |                     delete_line( hL );
      |                 end
      |                 add_line( MechSystem, [get_param( hAPInports(i), 'Name' ), '/1'], [get_param( hActuatedPrismatics(i), 'Name' ), '/1'] );
      |             end
      |        elseif strcmp( MotionConfig, 'Motion' )
      |             set_param( MechSystem, 'Tag', 'Motion' );
      |             for i = 1:NMotors
      |                 o = get_param( hMotors(i), 'Object' );
      |                 o.MotorType = 'Motion';
      |                 set_param( hMotInports(i), 'Name', [MotNameRoot{i}, '_pva'] );
      |                 hP = get_param( hMotInports(i), 'PortHandles' );
      |                 hL = get_param( hP.Outport, 'Line' );
      |                 if hL ~= -1
      |                     delete_line( hL );
      |                 end
      |                 add_line( MechSystem, [get_param( hMotInports(i), 'Name' ), '/1'], [get_param( hMotors(i), 'Name' ), '/1'] );
      |             end
      |             for i = 1:NActuators
      |                 o = get_param( hActuators(i), 'Object' );
      |                 o.ActuationType = 'Motion';
      |                 set_param( hActInports(i), 'Name', [ActNameRoot{i}, '_pva'] );
      |                 hP = get_param( hActInports(i), 'PortHandles' );
      |                 hL = get_param( hP.Outport, 'Line' );
      |                 if hL ~= -1
      |                     delete_line( hL );
      |                 end
      |                 add_line( MechSystem, [get_param( hActInports(i), 'Name' ), '/1'], [get_param( hActuators(i), 'Name' ), '/1'] );
      |             end
      |             for i = 1:NActuatedPrismatics
      |                 o = get_param( hActuatedPrismatics(i), 'Object' );
      |                 o.ActuationType = 'Motion';
      |                 set_param( hAPInports(i), 'Name', [APNameRoot{i}, '_pva'] );
      |                 hP = get_param( hAPInports(i), 'PortHandles' );
      |                 hL = get_param( hP.Outport, 'Line' );
      |                 if hL ~= -1
      |                     delete_line( hL );
      |                 end
      |                 add_line( MechSystem, [get_param( hAPInports(i), 'Name' ), '/1'], [get_param( hActuatedPrismatics(i), 'Name' ), '/1'] );
      |             end
      |         end
      |     elseif strcmp( MotionConfig, 'Inverse' )
      |        set_param( MechSystem, 'Tag', 'Inverse' );
      |        Inports = find_system(MechSystem,'LookUnderMasks','all','Tag','MechSystemMotorInport');
      |        for i = 1:NMotors
      |             hP = get_param( Inports{i}, 'PortHandles' );
      |             hL = get_param( hP.Outport, 'Line' );
      |             delete_line( hL );
      |             delete_block( Inports{i} );
      |             o = get_param( hMotors(i), 'Object' );
      |             o.MotorType = 'Inverse';
      |        end
      |        Inports = find_system(MechSystem,'LookUnderMasks','all','Tag','MechSystemActuatorInport');
      |        for i = 1:NActuators
      |             hP = get_param( Inports{i}, 'PortHandles' );
      |             hL = get_param( hP.Outport, 'Line' );
      |             delete_line( hL );
      |             delete_block( Inports{i} );
      |             o = get_param( hActuators(i), 'Object' );
      |             o.ActuatorType = 'Inverse';
      |        end
      |        Inports = find_system(MechSystem,'LookUnderMasks','all','Tag','MechSystemAPInport');
      |        for i = 1:NActuatedPrismatics
      |             hP = get_param( Inports{i}, 'PortHandles' );
      |             hL = get_param( hP.Outport, 'Line' );
      |             delete_line( hL );
      |             delete_block( Inports{i} );
      |             o = get_param( hActuatedPrismatics(i), 'Object' );
      |             o.ActuatorType = 'Inverse';
      |        end
      |     end
      | end
      | clear( 'hMechSystem', 'hOutports', 'i', 'InportName', 'Inports', 'MotionConfig', 'Motors', 'NameLength', 'NameRoot', 'NMotors', 'Outports', 'hInports', 'hL', 'hMotors', 'hP', 'hpMotor', 'InPos', 'MechSystem', 'o', 'OutportName', 'OutPos', 'ActOutports', 'hMotInports', 'hMotOutports', 'MotNameRoot', 'MotOutports', 'NActuators', 'ActNameRoot', 'hActInports', 'hActOutports', 'hActuators', 'hpActuator', 'hpPrisJoint', 'hPrisJoint', 'PrisJointLC2Pos', 'APNameRoot', 'APOutports', 'hActuatedPrismatics', 'hAPInports', 'hAPOutports', 'hpActuatedPrismatic', 'NActuatedPrismatics' );
  MotorTypeLibrary : Subsystem
  Motor_x : Subsystem  Tag=Torque  mask{MotorType=Torque}
      mask prompts: MotorType "Motor Type"
      mask TypeOptions MotorType: Torque | Motion | Shaft | Inverse
      mask Callback MotorType:
      | maskStr = get_param( gcb, 'MotorType' );
      | MotorBlockHandle = gcbh;
      | MotorBlockSystemName = [get_param( MotorBlockHandle, 'Parent' ), '/', get_param( MotorBlockHandle, 'Name' )];
      | CurrentConfig = get_param( MotorBlockHandle, 'Tag' );
      | if ~strcmp( maskStr, CurrentConfig )
      |     hInport = find_system(MotorBlockHandle,'LookUnderMasks','all','SearchDepth','1','BlockType','Inport');
      |     if ~isempty( hInport )
      |         hPH = get_param( hInport, 'PortHandles' );
      |         PortPosition = get_param( hInport, 'Position' );
      |         PortPositionStringForSetParam = ['[', num2str( PortPosition(1) ), ', ', num2str( PortPosition(2) ), ', ', num2str( PortPosition(3) ), ', ', num2str( PortPosition(4) ), ']'];
      |         hLine = get_param( hPH.Outport, 'Line' );
      |         delete_block( hInport );
      |         delete( hLine );
      |     end
      |     hExternalPort = find_system(MotorBlockHandle,'LookUnderMasks','all','Name','MotorShaft');
      |     if ~isempty( hExternalPort )
      |         hPH = get_param( hExternalPort, 'PortHandles' );
      |         PortPosition = get_param( hExternalPort, 'Position' );
      |         PortPositionStringForSetParam = ['[', num2str( PortPosition(1) ), ', ', num2str( PortPosition(2) ), ', ', num2str( PortPosition(3) ), ', ', num2str( PortPosition(4) ), ']'];
      |         hLine = get_param( hPH.RConn, 'Line' );
      |         delete_block( hExternalPort );
      |         delete( hLine );
      |     end
      |     hMotorBlock = find_system(MotorBlockHandle,'LookUnderMasks','all','Tag','Motor');
      |     BlockPos = get_param( hMotorBlock, 'Position' );
      |     MotorPositionStringForSetParam = ['[', num2str( BlockPos(1) ), ', ', num2str( BlockPos(2) ), ', ', num2str( BlockPos(3) ), ', ', num2str( BlockPos(4) ), ']'];
      |     delete_block( hMotorBlock );
      | 
      |     if strcmpi(maskStr, 'Torque')
      |         hMotorBlock = add_block( 'TerryBodyBlockLib2G/MotorTypeLibrary/TorqueMotor', [MotorBlockSystemName, '/TorqueMotor'] );
      |         set_param( hMotorBlock, 'LinkStatus', 'none' );
      |         set_param( MotorBlockHandle, 'Tag', 'Torque' );
      |         set_param( hMotorBlock, 'Position', MotorPositionStringForSetParam );
      |         hInport = add_block( 'simulink/Sources/In1', [MotorBlockSystemName, '/Torque(N*m)'] );
      |         set_param( hInport, 'Position', PortPositionStringForSetParam );
      |         hInportHandles = get_param( hInport, 'PortHandles' );
      |         hMotorPortHandles = get_param( hMotorBlock, 'PortHandles' );
      |         add_line(MotorBlockSystemName,hInportHandles.Outport(1),hMotorPortHandles.Inport(1));
      |     elseif strcmpi(maskStr, 'Motion')
      |         hMotorBlock = add_block( 'TerryBodyBlockLib2G/MotorTypeLibrary/MotionMotor', [MotorBlockSystemName, '/MotionMotor'] );
      |         set_param( hMotorBlock, 'LinkStatus', 'none' );
      |         set_param( MotorBlockHandle, 'Tag', 'Motion' );
      |         set_param( hMotorBlock, 'Position', MotorPositionStringForSetParam );
      |         hInport = add_block( 'simulink/Sources/In1', [MotorBlockSystemName, '/Motion( pva, deg, s )'] );
      |         set_param( hInport, 'Position', PortPositionStringForSetParam );
      |         hInportHandles = get_param( hInport, 'PortHandles' );
      |         hMotorPortHandles = get_param( hMotorBlock, 'PortHandles' );
      |         add_line(MotorBlockSystemName,hInportHandles.Outport(1),hMotorPortHandles.Inport(1));
      |     elseif strcmpi(maskStr, 'Shaft')
      |         hMotorBlock = add_block( 'TerryBodyBlockLib2G/MotorTypeLibrary/ShaftMotor', [MotorBlockSystemName, '/ShaftMotor'] );
      |         set_param( hMotorBlock, 'LinkStatus', 'none' );
      |         set_param( MotorBlockHandle, 'Tag', 'Shaft' );
      |         set_param( hMotorBlock, 'Position', MotorPositionStringForSetParam );
      |         hExternalPort = add_block( 'nesl_utility/Connection Port', [MotorBlockSystemName, '/MotorShaft'] );
      |         set_param( hExternalPort, 'Port', '1' );
      |         set_param( hExternalPort, 'Side', 'Left' );
      |         set_param( hExternalPort, 'Position', PortPositionStringForSetParam );
      |         hExPortHandles = get_param( hExternalPort, 'PortHandles' );
      |         hMotorPortHandles = get_param( hMotorBlock, 'PortHandles' );
      |         add_line(MotorBlockSystemName,hExPortHandles.RConn(1),hMotorPortHandles.LConn(1));
      |     end
      | end
      | clear( 'BlockPos', 'CurrentConfig', 'hExPortHandles', 'hExternalPort', 'hInport', 'hInportHandles', 'hLine', 'hMotorBlock', 'hMotorPortHandles', 'hPH', 'maskStr', 'MotorBlockHandle', 'MotorBlockSystemName', 'MotorPositionStringForSetParam', 'PortPosition', 'PortPositionStringForSetParam' );
  Motor_y : Subsystem  Tag=Torque  mask{MotorType=Torque}
      mask prompts: MotorType "Motor Type"
      mask TypeOptions MotorType: Torque | Motion | Shaft | Inverse
      mask Callback MotorType:
      | maskStr = get_param( gcb, 'MotorType' );
      | MotorBlockHandle = gcbh;
      | MotorBlockSystemName = [get_param( MotorBlockHandle, 'Parent' ), '/', get_param( MotorBlockHandle, 'Name' )];
      | CurrentConfig = get_param( MotorBlockHandle, 'Tag' );
      | if ~strcmp( maskStr, CurrentConfig )
      |     hInport = find_system(MotorBlockHandle,'LookUnderMasks','all','SearchDepth','1','BlockType','Inport');
      |     if ~isempty( hInport )
      |         hPH = get_param( hInport, 'PortHandles' );
      |         PortPosition = get_param( hInport, 'Position' );
      |         PortPositionStringForSetParam = ['[', num2str( PortPosition(1) ), ', ', num2str( PortPosition(2) ), ', ', num2str( PortPosition(3) ), ', ', num2str( PortPosition(4) ), ']'];
      |         hLine = get_param( hPH.Outport, 'Line' );
      |         delete_block( hInport );
      |         delete( hLine );
      |     end
      |     hExternalPort = find_system(MotorBlockHandle,'LookUnderMasks','all','Name','MotorShaft');
      |     if ~isempty( hExternalPort )
      |         hPH = get_param( hExternalPort, 'PortHandles' );
      |         PortPosition = get_param( hExternalPort, 'Position' );
      |         PortPositionStringForSetParam = ['[', num2str( PortPosition(1) ), ', ', num2str( PortPosition(2) ), ', ', num2str( PortPosition(3) ), ', ', num2str( PortPosition(4) ), ']'];
      |         hLine = get_param( hPH.RConn, 'Line' );
      |         delete_block( hExternalPort );
      |         delete( hLine );
      |     end
      |     hMotorBlock = find_system(MotorBlockHandle,'LookUnderMasks','all','Tag','Motor');
      |     BlockPos = get_param( hMotorBlock, 'Position' );
      |     MotorPositionStringForSetParam = ['[', num2str( BlockPos(1) ), ', ', num2str( BlockPos(2) ), ', ', num2str( BlockPos(3) ), ', ', num2str( BlockPos(4) ), ']'];
      |     delete_block( hMotorBlock );
      | 
      |     if strcmpi(maskStr, 'Torque')
      |         hMotorBlock = add_block( 'TerryBodyBlockLib2G/MotorTypeLibrary/TorqueMotor', [MotorBlockSystemName, '/TorqueMotor'] );
      |         set_param( hMotorBlock, 'LinkStatus', 'none' );
      |         set_param( MotorBlockHandle, 'Tag', 'Torque' );
      |         set_param( hMotorBlock, 'Position', MotorPositionStringForSetParam );
      |         hInport = add_block( 'simulink/Sources/In1', [MotorBlockSystemName, '/Torque(N*m)'] );
      |         set_param( hInport, 'Position', PortPositionStringForSetParam );
      |         hInportHandles = get_param( hInport, 'PortHandles' );
      |         hMotorPortHandles = get_param( hMotorBlock, 'PortHandles' );
      |         add_line(MotorBlockSystemName,hInportHandles.Outport(1),hMotorPortHandles.Inport(1));
      |     elseif strcmpi(maskStr, 'Motion')
      |         hMotorBlock = add_block( 'TerryBodyBlockLib2G/MotorTypeLibrary/MotionMotor', [MotorBlockSystemName, '/MotionMotor'] );
      |         set_param( hMotorBlock, 'LinkStatus', 'none' );
      |         set_param( MotorBlockHandle, 'Tag', 'Motion' );
      |         set_param( hMotorBlock, 'Position', MotorPositionStringForSetParam );
      |         hInport = add_block( 'simulink/Sources/In1', [MotorBlockSystemName, '/Motion( pva, deg, s )'] );
      |         set_param( hInport, 'Position', PortPositionStringForSetParam );
      |         hInportHandles = get_param( hInport, 'PortHandles' );
      |         hMotorPortHandles = get_param( hMotorBlock, 'PortHandles' );
      |         add_line(MotorBlockSystemName,hInportHandles.Outport(1),hMotorPortHandles.Inport(1));
      |     elseif strcmpi(maskStr, 'Shaft')
      |         hMotorBlock = add_block( 'TerryBodyBlockLib2G/MotorTypeLibrary/ShaftMotor', [MotorBlockSystemName, '/ShaftMotor'] );
      |         set_param( hMotorBlock, 'LinkStatus', 'none' );
      |         set_param( MotorBlockHandle, 'Tag', 'Shaft' );
      |         set_param( hMotorBlock, 'Position', MotorPositionStringForSetParam );
      |         hExternalPort = add_block( 'nesl_utility/Connection Port', [MotorBlockSystemName, '/MotorShaft'] );
      |         set_param( hExternalPort, 'Port', '1' );
      |         set_param( hExternalPort, 'Side', 'Left' );
      |         set_param( hExternalPort, 'Position', PortPositionStringForSetParam );
      |         hExPortHandles = get_param( hExternalPort, 'PortHandles' );
      |         hMotorPortHandles = get_param( hMotorBlock, 'PortHandles' );
      |         add_line(MotorBlockSystemName,hExPortHandles.RConn(1),hMotorPortHandles.LConn(1));
      |     end
      | end
      | clear( 'BlockPos', 'CurrentConfig', 'hExPortHandles', 'hExternalPort', 'hInport', 'hInportHandles', 'hLine', 'hMotorBlock', 'hMotorPortHandles', 'hPH', 'maskStr', 'MotorBlockHandle', 'MotorBlockSystemName', 'MotorPositionStringForSetParam', 'PortPosition', 'PortPositionStringForSetParam' );
  Motor_z : Subsystem  Tag=Torque  mask{MotorType=Torque}
      mask prompts: MotorType "Motor Type"
      mask TypeOptions MotorType: Torque | Motion | Shaft | Inverse
      mask Callback MotorType:
      | maskStr = get_param( gcb, 'MotorType' );
      | MotorBlockHandle = gcbh;
      | MotorBlockSystemName = [get_param( MotorBlockHandle, 'Parent' ), '/', get_param( MotorBlockHandle, 'Name' )];
      | CurrentConfig = get_param( MotorBlockHandle, 'Tag' );
      | if ~strcmp( maskStr, CurrentConfig )
      |     hInport = find_system(MotorBlockHandle,'LookUnderMasks','all','SearchDepth','1','BlockType','Inport');
      |     if ~isempty( hInport )
      |         hPH = get_param( hInport, 'PortHandles' );
      |         PortPosition = get_param( hInport, 'Position' );
      |         PortPositionStringForSetParam = ['[', num2str( PortPosition(1) ), ', ', num2str( PortPosition(2) ), ', ', num2str( PortPosition(3) ), ', ', num2str( PortPosition(4) ), ']'];
      |         hLine = get_param( hPH.Outport, 'Line' );
      |         delete_block( hInport );
      |         delete( hLine );
      |     end
      |     hExternalPort = find_system(MotorBlockHandle,'LookUnderMasks','all','Name','MotorShaft');
      |     if ~isempty( hExternalPort )
      |         hPH = get_param( hExternalPort, 'PortHandles' );
      |         PortPosition = get_param( hExternalPort, 'Position' );
      |         PortPositionStringForSetParam = ['[', num2str( PortPosition(1) ), ', ', num2str( PortPosition(2) ), ', ', num2str( PortPosition(3) ), ', ', num2str( PortPosition(4) ), ']'];
      |         hLine = get_param( hPH.RConn, 'Line' );
      |         delete_block( hExternalPort );
      |         delete( hLine );
      |     end
      |     hMotorBlock = find_system(MotorBlockHandle,'LookUnderMasks','all','Tag','Motor');
      |     BlockPos = get_param( hMotorBlock, 'Position' );
      |     MotorPositionStringForSetParam = ['[', num2str( BlockPos(1) ), ', ', num2str( BlockPos(2) ), ', ', num2str( BlockPos(3) ), ', ', num2str( BlockPos(4) ), ']'];
      |     delete_block( hMotorBlock );
      | 
      |     if strcmpi(maskStr, 'Torque')
      |         hMotorBlock = add_block( 'TerryBodyBlockLib2G/MotorTypeLibrary/TorqueMotor', [MotorBlockSystemName, '/TorqueMotor'] );
      |         set_param( hMotorBlock, 'LinkStatus', 'none' );
      |         set_param( MotorBlockHandle, 'Tag', 'Torque' );
      |         set_param( hMotorBlock, 'Position', MotorPositionStringForSetParam );
      |         hInport = add_block( 'simulink/Sources/In1', [MotorBlockSystemName, '/Torque(N*m)'] );
      |         set_param( hInport, 'Position', PortPositionStringForSetParam );
      |         hInportHandles = get_param( hInport, 'PortHandles' );
      |         hMotorPortHandles = get_param( hMotorBlock, 'PortHandles' );
      |         add_line(MotorBlockSystemName,hInportHandles.Outport(1),hMotorPortHandles.Inport(1));
      |     elseif strcmpi(maskStr, 'Motion')
      |         hMotorBlock = add_block( 'TerryBodyBlockLib2G/MotorTypeLibrary/MotionMotor', [MotorBlockSystemName, '/MotionMotor'] );
      |         set_param( hMotorBlock, 'LinkStatus', 'none' );
      |         set_param( MotorBlockHandle, 'Tag', 'Motion' );
      |         set_param( hMotorBlock, 'Position', MotorPositionStringForSetParam );
      |         hInport = add_block( 'simulink/Sources/In1', [MotorBlockSystemName, '/Motion( pva, deg, s )'] );
      |         set_param( hInport, 'Position', PortPositionStringForSetParam );
      |         hInportHandles = get_param( hInport, 'PortHandles' );
      |         hMotorPortHandles = get_param( hMotorBlock, 'PortHandles' );
      |         add_line(MotorBlockSystemName,hInportHandles.Outport(1),hMotorPortHandles.Inport(1));
      |     elseif strcmpi(maskStr, 'Shaft')
      |         hMotorBlock = add_block( 'TerryBodyBlockLib2G/MotorTypeLibrary/ShaftMotor', [MotorBlockSystemName, '/ShaftMotor'] );
      |         set_param( hMotorBlock, 'LinkStatus', 'none' );
      |         set_param( MotorBlockHandle, 'Tag', 'Shaft' );
      |         set_param( hMotorBlock, 'Position', MotorPositionStringForSetParam );
      |         hExternalPort = add_block( 'nesl_utility/Connection Port', [MotorBlockSystemName, '/MotorShaft'] );
      |         set_param( hExternalPort, 'Port', '1' );
      |         set_param( hExternalPort, 'Side', 'Left' );
      |         set_param( hExternalPort, 'Position', PortPositionStringForSetParam );
      |         hExPortHandles = get_param( hExternalPort, 'PortHandles' );
      |         hMotorPortHandles = get_param( hMotorBlock, 'PortHandles' );
      |         add_line(MotorBlockSystemName,hExPortHandles.RConn(1),hMotorPortHandles.LConn(1));
      |     end
      | end
      | clear( 'BlockPos', 'CurrentConfig', 'hExPortHandles', 'hExternalPort', 'hInport', 'hInportHandles', 'hLine', 'hMotorBlock', 'hMotorPortHandles', 'hPH', 'maskStr', 'MotorBlockHandle', 'MotorBlockSystemName', 'MotorPositionStringForSetParam', 'PortPosition', 'PortPositionStringForSetParam' );
  Px : Subsystem  mask(Prismatic X){}
      mask help: Prismatic Joint that constrains translation between two frames to occur only in the direction of their aligned x-axes.
  Pxy : Subsystem  mask(Prismatic X){}
      mask help: Prismatic Joint that constrains translation between two frames to occur only in the direction of their aligned x-axes.
  Py : Subsystem  mask(Prismatic Y){}
      mask help: Prismatic Joint that constrains translation between two frames to occur only in the direction of their aligned y-axes.
  Rx : Subsystem  mask(Revolute X){}
      mask help: Revolute Joint that constrains rotation between two frames to occur only about their aligned x-axes.
  Ry : Subsystem  mask(Revolute Y){}
      mask help: Revolute Joint that constrains rotation between two frames to occur only about their aligned y-axes.
  RzPx : Subsystem  mask(RzPx){}
      mask help: Rotational connection for aligned Z-axes on the Rz port. Prismatic connection for aligned X-axes on the Px port.
  SWForceActuator : Subsystem
  SWRope : Subsystem  mask{Rope_Length=0.7223487, Spring_Constant=1e5, Damping_Constant=1e3}
      mask prompts: Rope_Length "Rope Length (m)"; Spring_Constant "Spring Constant (N/m)"; Damping_Constant "Damping Constant (N.s/m)"
  SWSeparator : Subsystem  mask{Separator_Length=0.75, Spring_Constant=1e5, Damping_Constant=1e3}
      mask prompts: Separator_Length "Separator Length (m)"; Spring_Constant "Spring Constant (N/m)"; Damping_Constant "Damping Constant (N.s/m)"
  "World, Solver & Mech Settings" : Subsystem
